simulink model "u2dd_sl"  (R2023a)
settings: Solver=VariableStepAuto  StartTime=0.0  StopTime=10.0  RelTol=1e-3
settings Model: Creator=Boss  LastModifiedBy=Boss

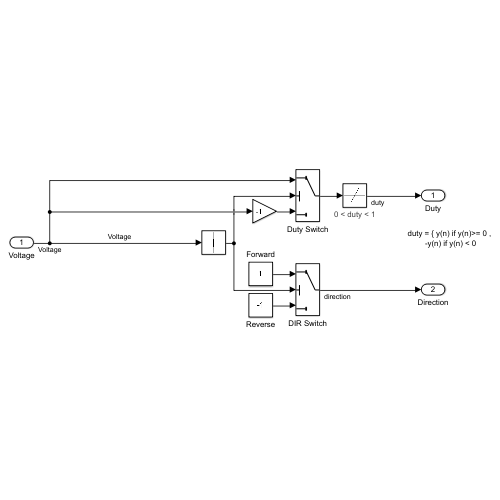
[thumbnail: Simulink's stored preview of the top-level diagram]
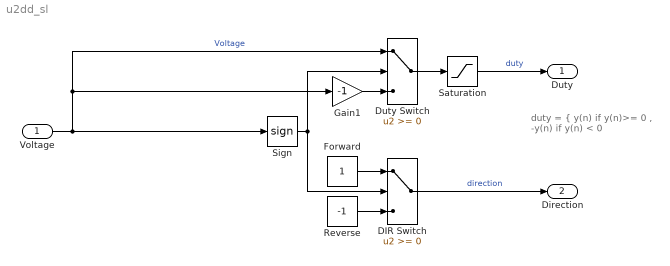
== system u2dd_sl ==
  note: duty = { y(n) if y(n)>= 0 ,
      |  -y(n) if y(n) < 0
  Voltage : Inport
  DIR Switch : Switch  SaturateOnIntegerOverflow=off  InputSameDT=off
  Duty Switch : Switch  SaturateOnIntegerOverflow=off  InputSameDT=off
  Forward : Constant  OutDataTypeStr=double
  Gain1 : Gain  Gain=-1
  Reverse : Constant  Value=-1  OutDataTypeStr=double
  Saturation : Saturate  UpperLimit=1  LowerLimit=0
      settings: AttributesFormatString=%<LowerLimit> < duty < %<UpperLimit>
  Sign : Signum
  Duty : Outport
  Direction : Outport  Port=2
  wires:
  Voltage/1 -> Sign/1, Gain1/1, Duty Switch/1  "Voltage"
  Forward/1 -> DIR Switch/1
  Reverse/1 -> DIR Switch/3
  Sign/1 -> Duty Switch/2, DIR Switch/2
  Gain1/1 -> Duty Switch/3
  DIR Switch/1 -> Direction/1  "direction"
  Duty Switch/1 -> Saturation/1
  Saturation/1 -> Duty/1  "duty"
